simulink model "InvertedPendulum_Simulink"  (R2023a)
settings: Solver=VariableStepAuto  StartTime=0.0  StopTime=60  RelTol=1e-3
libraries: dspsrcs4 x1, slpidlib x1, simulink x1
settings Model: Creator=ark19001  LastModifiedBy=ark19001
settings DebuggingCC: AlgebraicLoopMsg=none

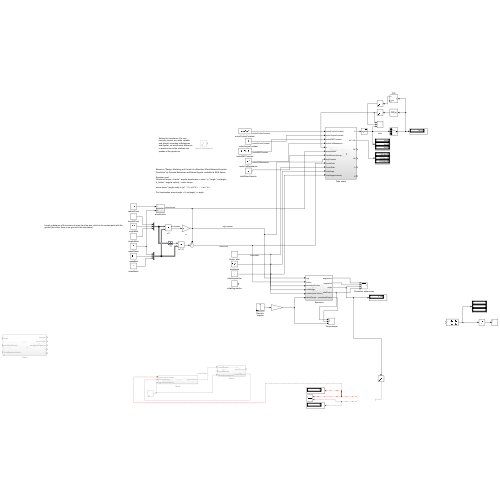
[thumbnail: Simulink's stored preview of the top-level diagram]
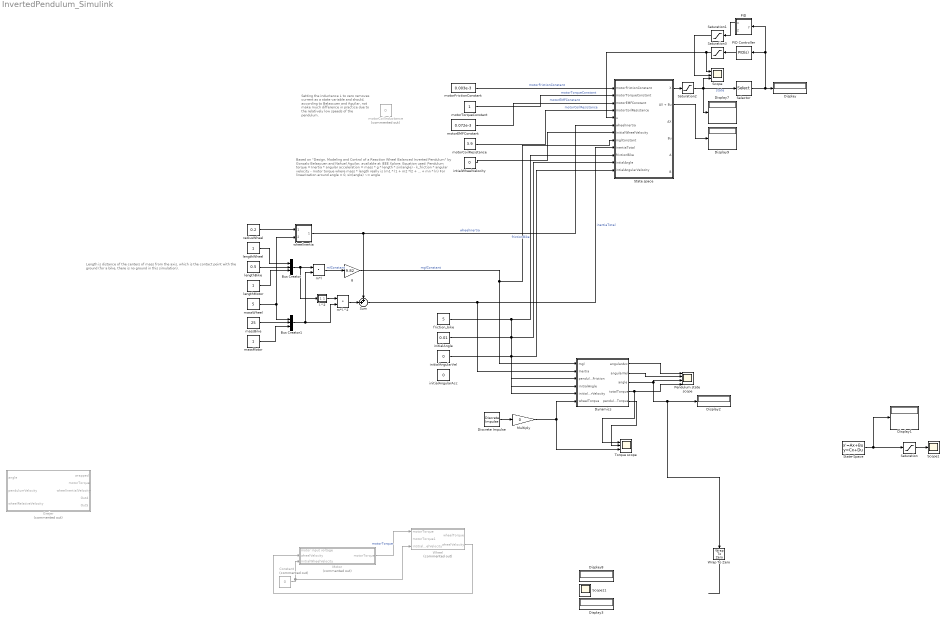
== system InvertedPendulum_Simulink ==
  note: Setting the inductance L to zero
      | removes current as a state variable
      | and should, according to Belascuen
      | and Aguilar, not make much difference
      | in practice due to the relatively low
      | speeds of the pendulum.
  note: Length is distance of the centers of mass from the axis, which is the contact point with the ground (for a bike, there is no ground in this simulation).
  note: Based on "Design, Modeling and Control of a Reaction Wheel Balanced Inverted Pendulum" by Gonzalo Belascuen and Nahuel Aguilar, available at IEEE Xplore.
      |
      | Equation used:
      | Pendulum torque = Inertia * angular acceleration = mass * g * length * sin(angle) - k_friction * angular velocity - motor torque
      |
      | where mass * length really is (m1 * l1 + m2 *l2 + ... + mn * ln)
      |
      | For linearization around angle = 0, sin(angle) ~= angle
  Bus Creator : BusCreator  Inputs=3
  Bus Creator1 : BusCreator  Inputs=3
  Constant : Constant  Commented=on  Value=0
  Discrete Impulse : dspsrcs4/Discrete  Impulse  Delay=1  SampleTime=1  FrameSample=1  OutputFrames=off  dataType=double  isSigned=on  wordLen=16  udDataType=sfix(16)  fracBitsMode=Best precision  numFracBits=15  OutDataTypeStr=double  LastOutDataTypeStr=double
  Display{,1..3,7..9} (7 alike) : Display
  Dynamics : Subsystem
  Grejer : Subsystem  Commented=on
  Motor : Subsystem  Commented=on
  Multiply : Gain  Gain=0
  PID : Subsystem  mask{P=3791.83003924061, I=3.69278957674571, D=0, ref=0, outputSign=-1}
      mask prompts: ref "Reference"; outputSign "Output sign"
      mask TypeOptions outputSign: -1 | 1
  PID Controller : slpidlib/PID Controller  Controller=PID  Form=Parallel  TimeDomain=Continuous-time  UseExternalTs=off  SampleTime=-1  IntegratorMethod=Forward Euler  FilterMethod=Forward Euler  ControllerParametersSource=internal  P=612.427466941037  I=1.3296046270024  UseKiTs=off  D=15064.3047991936  N=0.0365908385923072  UseFilter=on  TunerSelectOption=Transfer Function Based (PID Tuner App)  InitialConditionSource=internal  InitialConditionForIntegrator=0  InitialConditionForFilter=0  DifferentiatorICPrevScaledInput=0  ExternalReset=none  TrackingMode=off  Kt=1  LimitOutput=off  SatLimitsSource=internal  UpperSaturationLimit=inf  LowerSaturationLimit=-inf  LinearizeAsGain=on  AntiWindupMode=none  Kb=1  LimitIntegrator=off  UpperIntegratorSaturationLimit=inf  LowerIntegratorSaturationLimit=-inf  POutMin=[]  POutMax=[]  IOutMin=[]  IOutMax=[]  DOutMin=[]  DOutMax=[]  NOutMin=[]  NOutMax=[]  SumOutMin=[]  SumOutMax=[]  SaturationOutMin=[]  SaturationOutMax=[]  PParamMin=[]  PParamMax=[]  IParamMin=[]  IParamMax=[]  DParamMin=[]  DParamMax=[]  NParamMin=[]  NParamMax=[]  KbParamMin=[]  KbParamMax=[]  KtParamMin=[]  KtParamMax=[]  KbOutMin=[]  KbOutMax=[]  KtOutMin=[]  KtOutMax=[]  IntegratorOutMin=[]  IntegratorOutMax=[]  FilterOutMin=[]  FilterOutMax=[]  SumI1OutMin=[]  SumI1OutMax=[]  SumI2OutMin=[]  SumI2OutMax=[]  SumI3OutMin=[]  SumI3OutMax=[]  SumI4OutMin=[]  SumI4OutMax=[]  SumDOutMin=[]  SumDOutMax=[]  DifferentiatorOutMin=[]  DifferentiatorOutMax=[]  FilterDiffOutCoefMin=[]  FilterDiffOutCoefMax=[]  ReciprocalOutMin=[]  ReciprocalOutMax=[]  SumDenOutMin=[]  SumDenOutMax=[]  SumNumOutMin=[]  SumNumOutMax=[]  DivideOutMin=[]  DivideOutMax=[]  UdiffTsProdOutMin=[]  UdiffTsProdOutMax=[]  NTsProdOutMin=[]  NTsProdOutMax=[]  UintegralTsProdOutMin=[]  UintegralTsProdOutMax=[]  UngainTsProdOutMin=[]  UngainTsProdOutMax=[]  ClampingZeroOutDataTypeStr=Inherit: Inherit via back propagation  ClampingZeroOutMin=[]  ClampingZeroOutMax=[]  FilterDenConstantOutDataTypeStr=Inherit: Inherit via back propagation  FilterDenConstantOutMin=[]  FilterDenConstantOutMax=[]  PCopyOutDataTypeStr=Inherit: Inherit via back propagation  PCopyOutMin=[]  PCopyOutMax=[]  NCopyOutDataTypeStr=Inherit: Inherit via back propagation  NCopyOutMin=[]  NCopyOutMax=[]  IntegratorContinuousStateAttributes=''  IntegratorStateMustResolveToSignalObject=off  IntegratorRTWStateStorageClass=Auto  FilterContinuousStateAttributes=''  FilterStateMustResolveToSignalObject=off  FilterRTWStateStorageClass=Auto  ParallelPVariant=InternalParameters  IdealPVariant=Disabled  IVariant=InternalParameters  DVariant=InternalParameters  IntegratorVariant=Continuous  SatVariant=Disabled  AWVariant=Passthrough  PCopyVariant=Disabled  TRVariant=Disabled  FdbkBlocksVariant=Forward  IdealPFdbkVariant=Disabled  SatFdbkVariant=Disabled  DerivativeFilterVariant=ContFilter  NVariant=InternalParameters  NCopyVariant=Disabled  FilterICVariant=InternalICsFilter  IntegratorICVariant=InternalICs  ExternalResetVariant=Disabled  TRSumVariant=Passthrough  SumFdbkVariant=Disabled  SumVariant=Sum_PID  TsampFilterVariant=InternalTs  TsampNgainVariant=Passthrough  TsampIntegralVariant=Disabled_SignalSpec  ExternalSaturationOutDataTypeStr=Inherit: Same as second input
  Pendulum state scope : Scope  NumInputPorts=4
  Saturation : Saturate  UpperLimit=1000  LowerLimit=-1000
  Saturation1 : Saturate  UpperLimit=24  LowerLimit=-24
  Saturation2 : Saturate  UpperLimit=10000  LowerLimit=-10000
  Saturation3 : Saturate  UpperLimit=24  LowerLimit=-24
  Scope : Scope  NumInputPorts=3
  Scope1 : Scope
  Scope11 : Scope  NumInputPorts=2
  Selector : Selector  InputPortWidth=3  IndexOptions=Index vector (dialog)  Indices=1  OutputSizes=1
  State space : Subsystem
  State-Space : StateSpace  A=[0 1 0; 14.59 0.4016 0.08032; -14.59 -0.4016 -5.08]  B=[0;-0.0206;1.303]  C=eye(3)  D=[0;0;0]  InitialCondition=[0.00;0;0]
  Sum : Sum  Inputs=++|
  Torque scope : Scope  NumInputPorts=3
  Wheel : Subsystem  Commented=on
  Wrap To Zero : simulink/Discontinuities/Wrap To Zero  Threshold=2*pi
  friction_bike : Constant  Value=5
  g : Gain  Gain=9.82
  initialAngle : Constant  Value=0.01
  initialAngularAcc : Constant  Value=0
  initialAngularVel : Constant  Value=0
  intialWheelVelocity : Constant  Value=0
  l.^2 : MATLAB Function  TreatAsAtomicUnit=on
  lengthBike : Constant  Value=0.5
  lengthMotor : Constant
  lengthWheel : Constant
  m*l : DotProduct  OutDataTypeStr=Inherit: Inherit via internal rule
  m*l.^2 : DotProduct  OutDataTypeStr=Inherit: Inherit via internal rule
  massBike : Constant  Value=25
  massMotor : Constant
  massWheel : Constant  Value=5
  motorCoilInductance : Constant  Commented=on  Value=0
  motorCoilResistance : Constant  Value=3.9
  motorEMFConstant : Constant  Value=0.072e-3
  motorFrictionConstant : Constant  Value=0.003e-3
  motorTorqueConstant : Constant
  radiusWheel : Constant  Value=0.2
  wheelInertia : Subsystem
  wires:
  massWheel/1 -> Bus Creator1/1, wheelInertia/2(In2)
  friction_bike/1 -> State space/10(frictionBike), Dynamics/3(pendulumFriction)  "frictionBike"
  initialAngle/1 -> State space/11(intialAngle), Dynamics/4(initialAngle)
  initialAngularVel/1 -> State space/12(intialAngularVelocity), Dynamics/5(initialAngularVelocity)
  m*l/1 -> g/1  "mlConstant"
  radiusWheel/1 -> wheelInertia/1(In1)
  motorFrictionConstant/1 -> State space/1(motorFrictionConstant)  "motorFrictionConstant"
  motorTorqueConstant/1 -> State space/2(motorTorqueConstant)  "motorTorqueConstant"
  motorEMFConstant/1 -> State space/3(motorEMFConstant)  "motorEMFConstant"
  motorCoilResistance/1 -> State space/4(motorCoilResistance)  "motorCoilResistance"
  wheelInertia/1(wheelInertia) -> State space/6(wheelInertia), Sum/1  "wheelInertia"
  intialWheelVelocity/1 -> State space/7(initialWheelVelocity)
  State-Space/1 -> Display1/1, Saturation/1
  ? -> Display3/1, Scope11/2
  ? -> Scope11/1, Motor/1(motor input voltage), Display8/1
  Wrap To Zero/1 -> ?
  Dynamics/1(angularAcc) -> Pendulum state scope/1
  Dynamics/2(angularVel) -> Pendulum state scope/2
  Dynamics/3(angle) -> Display2/1, Wrap To Zero/1, Pendulum state scope/3
  Dynamics/4(totalTorque) -> Torque scope/1, Pendulum state scope/4
  Dynamics/5(pendulumTorque) -> Torque scope/2
  Motor/1(motorTorque) -> Wheel/1(motorTorque)  "motorTorque"
  Constant/1 -> Motor/3(initialWheelVelocity), Wheel/3(intitialWheelVelocity)
  Wheel/2(wheelVelocity) -> Motor/2(wheelVelocity)
  Discrete Impulse/1 -> Multiply/1
  Multiply/1 -> Torque scope/3, Dynamics/6(wheelTorque)
  massBike/1 -> Bus Creator1/2
  massMotor/1 -> Bus Creator1/3
  lengthMotor/1 -> Bus Creator/3
  Bus Creator/1 -> l.^2/1(u), m*l/1
  Bus Creator1/1 -> m*l.^2/2, m*l/2
  lengthBike/1 -> Bus Creator/2
  lengthWheel/1 -> Bus Creator/1
  g/1 -> State space/8(mglConstant), Dynamics/1(mgl)  "mglConstant"
  l.^2/1(y) -> m*l.^2/1
  m*l.^2/1 -> Sum/2
  Sum/1 -> State space/9(inertiaTotal), Dynamics/2(Inertia)  "inertiaTotal"
  Saturation/1 -> Scope1/1
  State space/1(X) -> Saturation2/1
  State space/2(AX + Bu) -> Display9/1
  Selector/1 -> Display/1, PID Controller/1, PID/1(y)
  Saturation2/1 -> Display7/1, Scope/3, Selector/1  "state"
  PID/1(u) -> Saturation1/1
  Saturation1/1 -> Scope/2
  PID Controller/1 -> Saturation3/1
  Saturation3/1 -> State space/5(u), Scope/1

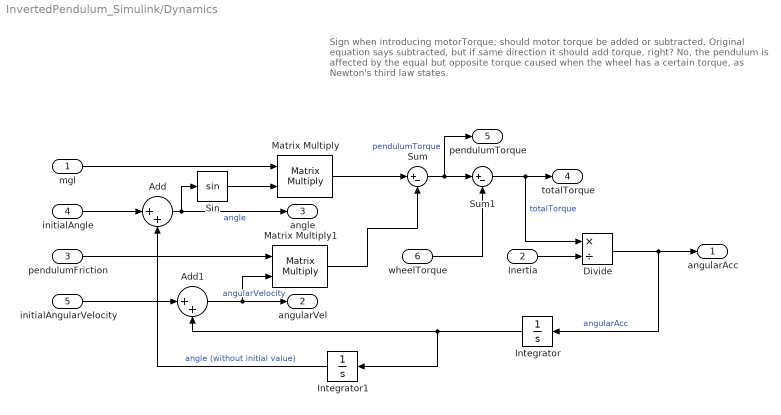
== system InvertedPendulum_Simulink/Dynamics ==
  note: Sign when introducing motorTorque; should motor torque be added or subtracted. Original equation says subtracted, but if same direction it should add torque, right? No, the pendulum is affected by the equal but opposite torque caused when the wheel has a certain torque, as Newton's third law states.
  mgl : Inport
  Inertia : Inport  Port=2
  pendulumFriction : Inport  Port=3
  initialAngle : Inport  Port=4
  initialAngularVelocity : Inport  Port=5
  wheelTorque : Inport  Port=6
  Add : Sum  Inputs=|++
  Add1 : Sum  Inputs=|++
  Divide : Product  Inputs=*/
  Integrator : Integrator
  Integrator1 : Integrator
  Matrix Multiply : Product  Multiplication=Matrix(*)
  Matrix Multiply1 : Product  Multiplication=Matrix(*)
  Sin : Trigonometry
  Sum : Sum  Inputs=|+-
  Sum1 : Sum  Inputs=|+-
  angularAcc : Outport
  angularVel : Outport  Port=2
  angle : Outport  Port=3
  totalTorque : Outport  Port=4
  pendulumTorque : Outport  Port=5
  wires:
  Integrator/1 -> Add1/2, Integrator1/1
  Add/1 -> angle/1, Sin/1  "angle"
  Integrator1/1 -> Add/2  "angle (without initial value)"
  Divide/1 -> angularAcc/1, Integrator/1  "angularAcc"
  initialAngularVelocity/1 -> Add1/1
  initialAngle/1 -> Add/1
  mgl/1 -> Matrix Multiply/1
  Sin/1 -> Matrix Multiply/2
  pendulumFriction/1 -> Matrix Multiply1/1
  Add1/1 -> angularVel/1, Matrix Multiply1/2  "angularVelocity"
  Matrix Multiply/1 -> Sum/1
  Matrix Multiply1/1 -> Sum/2
  Sum/1 -> pendulumTorque/1, Sum1/1  "pendulumTorque"
  wheelTorque/1 -> Sum1/2
  Sum1/1 -> Divide/1, totalTorque/1  "totalTorque"
  Inertia/1 -> Divide/2

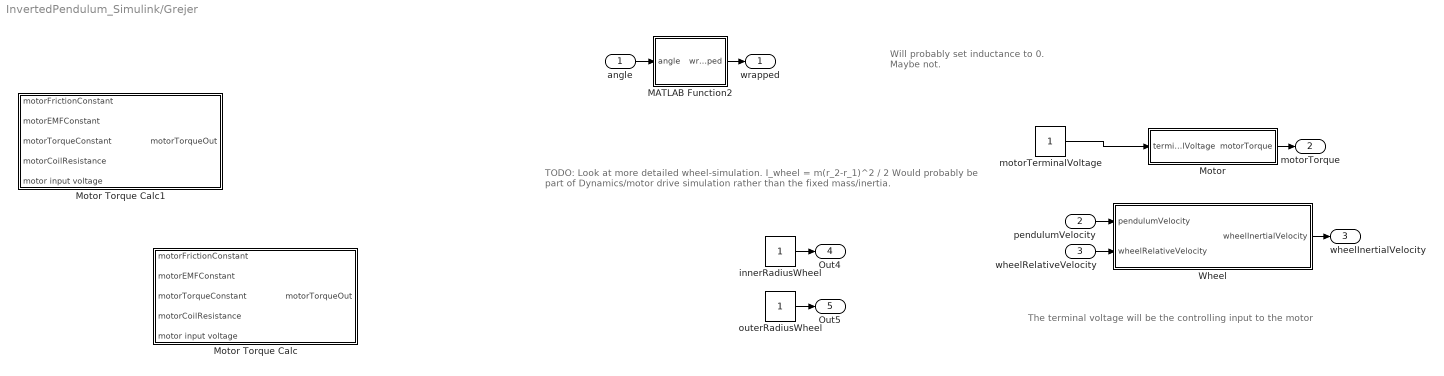
== system InvertedPendulum_Simulink/Grejer ==
  note: The terminal voltage will be the controlling input to the motor
  note: Will probably set inductance to 0.
      | Maybe not.
  note: TODO: Look at more detailed wheel-simulation. I_wheel = m(r_2-r_1)^2 / 2
      | Would probably be part of Dynamics/motor drive simulation rather than the fixed mass/inertia.
  angle : Inport
  pendulumVelocity : Inport  Port=2
  wheelRelativeVelocity : Inport  Port=3
  MATLAB Function2 : MATLAB Function  TreatAsAtomicUnit=on
  Motor : Subsystem
  Motor Torque Calc : Subsystem
  Motor Torque Calc1 : Subsystem
  Wheel : Subsystem
  innerRadiusWheel : Constant
  motorTerminalVoltage : Constant
  outerRadiusWheel : Constant
  wrapped : Outport
  motorTorque : Outport  Port=2
  wheelInertialVelocity : Outport  Port=3
  Out4 : Outport  Port=4
  Out5 : Outport  Port=5
  wires:
  outerRadiusWheel/1 -> Out5/1
  angle/1 -> MATLAB Function2/1(angle)
  pendulumVelocity/1 -> Wheel/1(pendulumVelocity)
  Motor/1(motorTorque) -> motorTorque/1
  motorTerminalVoltage/1 -> Motor/1(terminalVoltage)
  wheelRelativeVelocity/1 -> Wheel/2(wheelRelativeVelocity)
  Wheel/1(wheelInertialVelocity) -> wheelInertialVelocity/1
  MATLAB Function2/1(wrapped) -> wrapped/1
  innerRadiusWheel/1 -> Out4/1

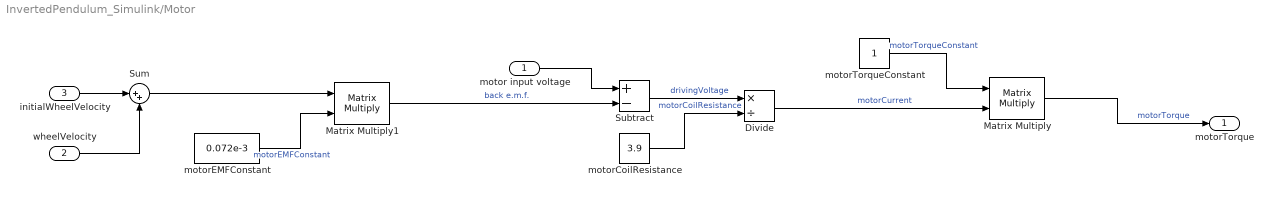
== system InvertedPendulum_Simulink/Motor ==
  motor input voltage : Inport
  wheelVelocity : Inport  Port=2
  initialWheelVelocity : Inport  Port=3
  Divide : Product  Inputs=*/
  Matrix Multiply : Product  Multiplication=Matrix(*)
  Matrix Multiply1 : Product  Multiplication=Matrix(*)
  Subtract : Sum  Inputs=+-
  Sum : Sum  Inputs=|++
  motorCoilResistance : Constant  Value=3.9
  motorEMFConstant : Constant  Value=0.072e-3
  motorTorqueConstant : Constant
  motorTorque : Outport
  wires:
  Matrix Multiply/1 -> motorTorque/1  "motorTorque"
  Divide/1 -> Matrix Multiply/2  "motorCurrent"
  motorTorqueConstant/1 -> Matrix Multiply/1  "motorTorqueConstant"
  motor input voltage/1 -> Subtract/1
  initialWheelVelocity/1 -> Sum/1
  motorEMFConstant/1 -> Matrix Multiply1/2  "motorEMFConstant"
  Matrix Multiply1/1 -> Subtract/2  "back e.m.f."
  Subtract/1 -> Divide/1  "drivingVoltage"
  Sum/1 -> Matrix Multiply1/1
  motorCoilResistance/1 -> Divide/2  "motorCoilResistance"
  wheelVelocity/1 -> Sum/2

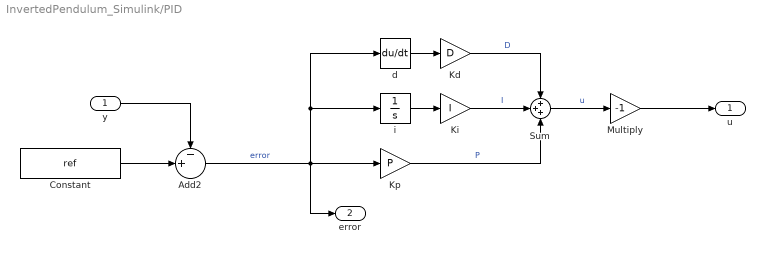
== system InvertedPendulum_Simulink/PID ==
  y : Inport
  Add2 : Sum  Inputs=-+|
  Constant : Constant  Value=ref
  Kd : Gain  Gain=D
  Ki : Gain  Gain=I
  Kp : Gain  Gain=P
  Multiply : Gain  Gain=-1
  Sum : Sum  Inputs=+++
  d : Derivative
  i : Integrator
  u : Outport
  error : Outport  Port=2
  wires:
  Add2/1 -> d/1, i/1, error/1, Kp/1  "error"
  d/1 -> Kd/1
  i/1 -> Ki/1
  Ki/1 -> Sum/2  "I"
  Kd/1 -> Sum/1  "D"
  Kp/1 -> Sum/3  "P"
  Constant/1 -> Add2/2
  y/1 -> Add2/1
  Sum/1 -> Multiply/1  "u"
  Multiply/1 -> u/1

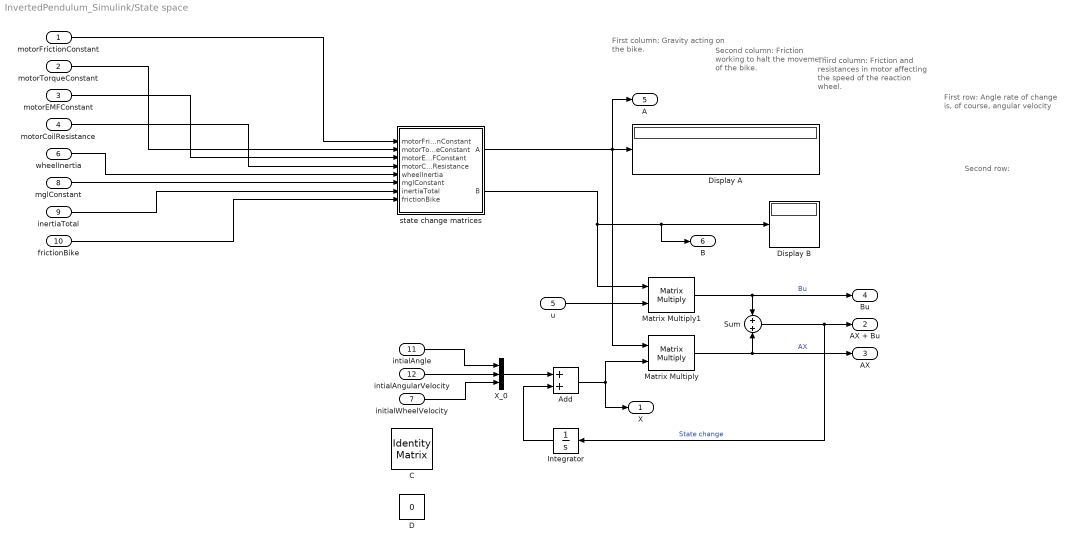
== system InvertedPendulum_Simulink/State space ==
  note: Second row:
  note: Second column:
      | Friction working to halt
      | the movement of the bike.
  note: Third column:
      | Friction and resistances in
      | motor affecting the speed
      | of the reaction wheel.
  note: First row:
      | Angle rate of change is,
      | of course, angular velocity
  note: First column:
      | Gravity acting on the bike.
  motorFrictionConstant : Inport
  motorTorqueConstant : Inport  Port=2
  motorEMFConstant : Inport  Port=3
  motorCoilResistance : Inport  Port=4
  u : Inport  Port=5
  wheelInertia : Inport  Port=6
  initialWheelVelocity : Inport  Port=7
  mglConstant : Inport  Port=8
  inertiaTotal : Inport  Port=9
  frictionBike : Inport  Port=10
  intialAngle : Inport  Port=11
  intialAngularVelocity : Inport  Port=12
  Add : Sum
  C : IdentityMatrix  OutputDimensions=3
  D : Constant  Value=0
  Display A : Display
  Display B : Display
  Integrator : Integrator
  Matrix Multiply : Product  Multiplication=Matrix(*)
  Matrix Multiply1 : Product  Multiplication=Matrix(*)
  Sum : Sum  Inputs=+|+
  X_0 : BusCreator  Inputs=3
  state change matrices : Subsystem
  X : Outport
  AX + Bu : Outport  Port=2
  AX : Outport  Port=3
  Bu : Outport  Port=4
  A : Outport  Port=5
  B : Outport  Port=6
  wires:
  u/1 -> Matrix Multiply1/2
  Add/1 -> X/1, Matrix Multiply/2
  X_0/1 -> Add/1
  Matrix Multiply/1 -> Sum/2, AX/1  "AX"
  Sum/1 -> AX + Bu/1, Integrator/1  "State change"
  Matrix Multiply1/1 -> Bu/1, Sum/1  "Bu"
  motorTorqueConstant/1 -> state change matrices/2(motorTorqueConstant)
  state change matrices/1(A) -> A/1, Matrix Multiply/1, Display A/1
  Integrator/1 -> Add/2
  state change matrices/2(B) -> B/1, Display B/1, Matrix Multiply1/1
  inertiaTotal/1 -> state change matrices/7(inertiaTotal)
  initialWheelVelocity/1 -> X_0/3
  intialAngle/1 -> X_0/1
  motorFrictionConstant/1 -> state change matrices/1(motorFrictionConstant)
  motorCoilResistance/1 -> state change matrices/4(motorCoilResistance)
  mglConstant/1 -> state change matrices/6(mglConstant)
  frictionBike/1 -> state change matrices/8(frictionBike)
  motorEMFConstant/1 -> state change matrices/3(motorEMFConstant)
  wheelInertia/1 -> state change matrices/5(wheelInertia)
  intialAngularVelocity/1 -> X_0/2

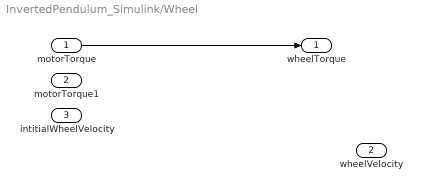
== system InvertedPendulum_Simulink/Wheel ==
  motorTorque : Inport
  motorTorque1 : Inport  Port=2
  intitialWheelVelocity : Inport  Port=3
  wheelTorque : Outport
  wheelVelocity : Outport  Port=2
  wires:
  motorTorque/1 -> wheelTorque/1

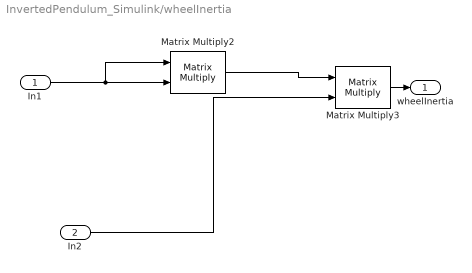
== system InvertedPendulum_Simulink/wheelInertia ==
  In1 : Inport
  In2 : Inport  Port=2
  Matrix Multiply2 : Product  Multiplication=Matrix(*)
  Matrix Multiply3 : Product  Multiplication=Matrix(*)
  wheelInertia : Outport
  wires:
  Matrix Multiply2/1 -> Matrix Multiply3/1
  In1/1 -> Matrix Multiply2/1, Matrix Multiply2/2
  Matrix Multiply3/1 -> wheelInertia/1
  In2/1 -> Matrix Multiply3/2

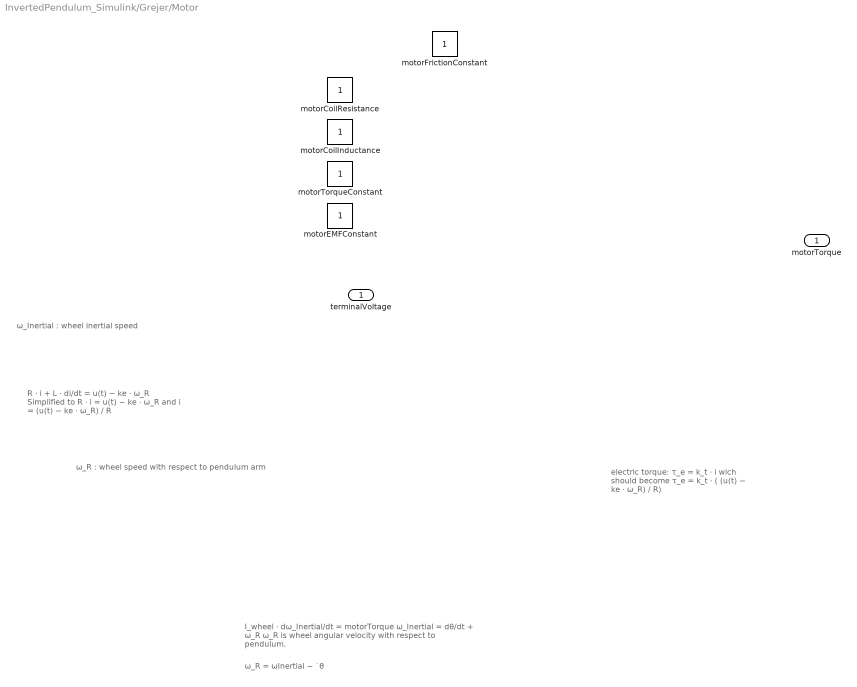
== system InvertedPendulum_Simulink/Grejer/Motor ==
  note: I_wheel · dω_Inertial/dt = motorTorque
      | ω_Inertial = dθ/dt + ω_R
      | ω_R is wheel angular velocity with respect to pendulum.
  note: electric torque:
      | τ_e = k_t · i
      | wich should become
      | τ_e = k_t · ( (u(t) − ke · ω_R) / R)
  note: ω_Inertial : wheel inertial speed
  note: ω_R : wheel speed with respect to pendulum arm
  note: ω_R = ωInertial − ˙θ
  note: R · i + L · di/dt = u(t) − ke · ω_R
      | Simplified to
      | R · i = u(t) − ke · ω_R and
      | i = (u(t) − ke · ω_R) / R
  terminalVoltage : Inport
  motorCoilInductance : Constant
  motorCoilResistance : Constant
  motorEMFConstant : Constant
  motorFrictionConstant : Constant
  motorTorqueConstant : Constant
  motorTorque : Outport

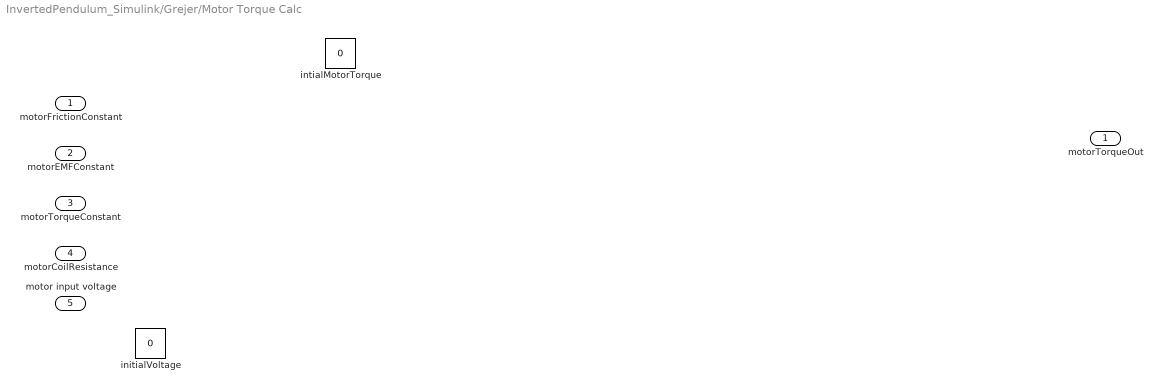
== system InvertedPendulum_Simulink/Grejer/Motor Torque Calc ==
  motorFrictionConstant : Inport
  motorEMFConstant : Inport  Port=2
  motorTorqueConstant : Inport  Port=3
  motorCoilResistance : Inport  Port=4
  motor input voltage : Inport  Port=5
  initialVoltage : Constant  Value=0
  intialMotorTorque : Constant  Value=0
  motorTorqueOut : Outport

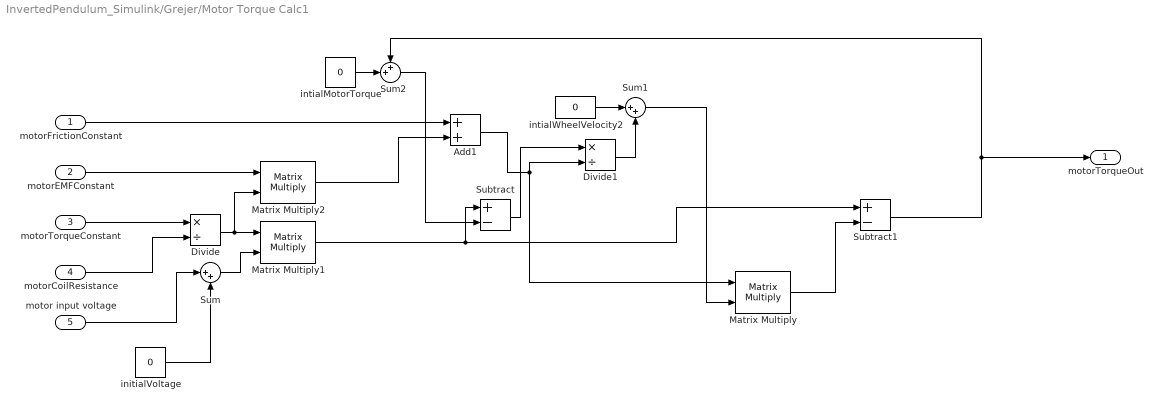
== system InvertedPendulum_Simulink/Grejer/Motor Torque Calc1 ==
  motorFrictionConstant : Inport
  motorEMFConstant : Inport  Port=2
  motorTorqueConstant : Inport  Port=3
  motorCoilResistance : Inport  Port=4
  motor input voltage : Inport  Port=5
  Add1 : Sum
  Divide : Product  Inputs=*/
  Divide1 : Product  Inputs=*/
  Matrix Multiply : Product  Multiplication=Matrix(*)
  Matrix Multiply1 : Product  Multiplication=Matrix(*)
  Matrix Multiply2 : Product  Multiplication=Matrix(*)
  Subtract : Sum  Inputs=+-
  Subtract1 : Sum  Inputs=+-
  Sum : Sum  Inputs=|++
  Sum1 : Sum  Inputs=|++
  Sum2 : Sum  Inputs=++|
  initialVoltage : Constant  Value=0
  intialMotorTorque : Constant  Value=0
  intialWheelVelocity2 : Constant  Value=0
  motorTorqueOut : Outport
  wires:
  Add1/1 -> Matrix Multiply/1, Divide1/2
  motorCoilResistance/1 -> Divide/2
  Divide1/1 -> Sum1/2
  Matrix Multiply2/1 -> Add1/2
  Divide/1 -> Matrix Multiply2/2, Matrix Multiply1/1
  intialWheelVelocity2/1 -> Sum1/1
  Matrix Multiply1/1 -> Subtract1/1, Subtract/1
  Subtract/1 -> Divide1/1
  Sum1/1 -> Matrix Multiply/2
  motorFrictionConstant/1 -> Add1/1
  motorTorqueConstant/1 -> Divide/1
  motorEMFConstant/1 -> Matrix Multiply2/1
  Matrix Multiply/1 -> Subtract1/2
  Subtract1/1 -> Sum2/1, motorTorqueOut/1
  Sum/1 -> Matrix Multiply1/2
  Sum2/1 -> Subtract/2
  intialMotorTorque/1 -> Sum2/2
  motor input voltage/1 -> Sum/1
  initialVoltage/1 -> Sum/2

== system InvertedPendulum_Simulink/Grejer/Wheel ==
  pendulumVelocity : Inport
  wheelRelativeVelocity : Inport  Port=2
  Add : Sum  Inputs=+++
  intialWheelVelocity : Constant  Value=0
  wheelInertialVelocity : Outport
  wires:
  wheelRelativeVelocity/1 -> Add/3
  intialWheelVelocity/1 -> Add/2
  Add/1 -> wheelInertialVelocity/1  "wheelInertialVelocity"
  pendulumVelocity/1 -> Add/1

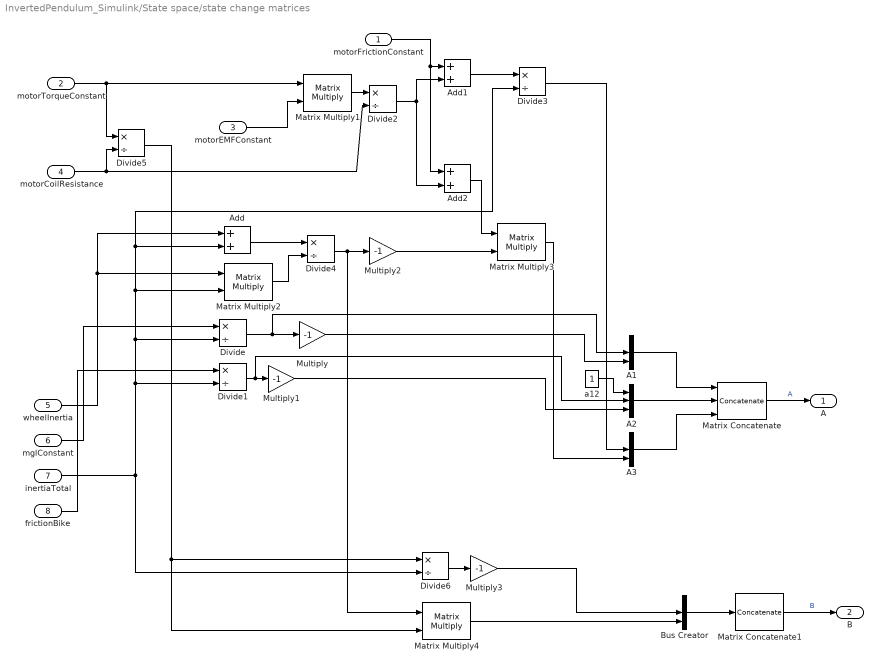
== system InvertedPendulum_Simulink/State space/state change matrices ==
  motorFrictionConstant : Inport
  motorTorqueConstant : Inport  Port=2
  motorEMFConstant : Inport  Port=3
  motorCoilResistance : Inport  Port=4
  wheelInertia : Inport  Port=5
  mglConstant : Inport  Port=6
  inertiaTotal : Inport  Port=7
  frictionBike : Inport  Port=8
  A1 : BusCreator  Inputs=3
  A2 : BusCreator  Inputs=3
  A3 : BusCreator  Inputs=3
  Add : Sum
  Add1 : Sum
  Add2 : Sum
  Bus Creator : BusCreator  Inputs=3
  Divide{,1..6} (7 alike) : Product  Inputs=*/
  Matrix Concatenate : Concatenate  NumInputs=3  Mode=Multidimensional array  ConcatenateDimension=2
  Matrix Concatenate1 : Concatenate  NumInputs=1  Mode=Multidimensional array  ConcatenateDimension=2
  Matrix Multiply{1..4} (4 alike) : Product  Multiplication=Matrix(*)
  Multiply{,1..3} (4 alike) : Gain  Gain=-1
  a12 : Constant
  A : Outport
  B : Outport  Port=2
  wires:
  Add/1 -> Divide4/1
  Multiply2/1 -> Matrix Multiply3/2
  A3/1 -> Matrix Concatenate/3
  motorEMFConstant/1 -> Matrix Multiply1/2
  Divide/1 -> A1/2, Multiply/1
  Matrix Concatenate/1 -> A/1  "A"
  motorCoilResistance/1 -> Divide2/2, Divide5/2
  inertiaTotal/1 -> Divide6/2, Matrix Multiply2/2, Divide3/2, Add/2, Divide/2, Divide1/2
  Divide1/1 -> A2/2, Multiply1/1
  frictionBike/1 -> Divide1/1
  Multiply1/1 -> A2/3
  A2/1 -> Matrix Concatenate/2
  Divide2/1 -> Add2/2, Add1/2
  Matrix Multiply3/1 -> A3/3
  a12/1 -> A2/1
  motorTorqueConstant/1 -> Matrix Multiply1/1, Divide5/1
  A1/1 -> Matrix Concatenate/1
  motorFrictionConstant/1 -> Add2/1, Add1/1
  mglConstant/1 -> Divide/1
  Multiply/1 -> A1/3
  Matrix Multiply2/1 -> Divide4/2
  Divide4/1 -> Matrix Multiply4/1, Multiply2/1
  wheelInertia/1 -> Matrix Multiply2/1, Add/1
  Matrix Multiply1/1 -> Divide2/1
  Divide3/1 -> A3/2
  Add2/1 -> Matrix Multiply3/1
  Add1/1 -> Divide3/1
  Bus Creator/1 -> Matrix Concatenate1/1
  Matrix Multiply4/1 -> Bus Creator/3
  Divide5/1 -> Matrix Multiply4/2, Divide6/1
  Divide6/1 -> Multiply3/1
  Multiply3/1 -> Bus Creator/2
  Matrix Concatenate1/1 -> B/1  "B"

== matlab function InvertedPendulum_Simulink/Grejer/MATLAB Function2 ==
  data: angle input; wrapped output
function wrapped = wrapAngle(angle)

wrapped= wrapToPi(angle);

== matlab function InvertedPendulum_Simulink/l.^2 ==
  data: u input; y output
function y = fcn(u)

y = u.^2;
